simulink model "20240109_HVDCMMCInterconnection"  (R2023b)
settings: Solver=FixedStepDiscrete  StartTime=0.0  StopTime=2  FixedStep=Ts_Power  RelTol=1e-4  EnableMultiTasking=on
PreLoadFcn:
  | HVDCMMCInterconnectionParam
StartFcn:
  | tic
StopFcn:
  | toc
values from neighbouring files (symbols this model uses):
  C_PM = 1.758e-3    (= 0.001758)    [HVDCMMCInterconnectionParam.m]
  Cg = 50e-9    (= 5e-08)    [HVDCMMCInterconnectionParam.m]
  D_R = 0.001    [HVDCMMCInterconnectionParam.m]
  D_Rs = 1e8    (= 100000000)    [HVDCMMCInterconnectionParam.m]
  D_Vf = 0    [HVDCMMCInterconnectionParam.m]
  Fnom = 50    [HVDCMMCInterconnectionParam.m]
  HRM = 2    [HVDCMMCInterconnectionParam.m]
  Ki_Ireg = 6    [HVDCMMCInterconnectionParam.m]
  Ki_Preg = 1.0    (= 1)    [HVDCMMCInterconnectionParam.m]
  Ki_Qreg = 1.0    (= 1)    [HVDCMMCInterconnectionParam.m]
  Ki_VDCreg = 100    [HVDCMMCInterconnectionParam.m]
  Kp_Ireg = 0.6    [HVDCMMCInterconnectionParam.m]
  Kp_Preg = 0.5/3    (= 0.166666666667)    [HVDCMMCInterconnectionParam.m]
  Kp_Qreg = 0.5/3    (= 0.166666666667)    [HVDCMMCInterconnectionParam.m]
  Kp_VDCreg = 4    [HVDCMMCInterconnectionParam.m]
  L_cable = 15e-3    (= 0.015)    [HVDCMMCInterconnectionParam.m]
  Larm = Larm_pu*(Zb_ac/(2*pi*Fnom))    [HVDCMMCInterconnectionParam.m]
  Lff = Larm_pu/2    (= 0.075)    [HVDCMMCInterconnectionParam.m]
  Limits_Ireg = [ 2.0  -2.0]    [HVDCMMCInterconnectionParam.m]
  Limits_Preg = [ 1.2, 0.8 ]    [HVDCMMCInterconnectionParam.m]
  Limits_Qreg = [ 0.25, -0.25 ]    [HVDCMMCInterconnectionParam.m]
  Limits_VDCreg = [ 2.0  -2.0]    [HVDCMMCInterconnectionParam.m]
  Lxfo = 0.12    [HVDCMMCInterconnectionParam.m]
  Nb_PM = 36    [HVDCMMCInterconnectionParam.m]
  Pnom = 1000e6    (= 1000000000)    [HVDCMMCInterconnectionParam.m]
  R_cable = 0.5    [HVDCMMCInterconnectionParam.m]
  R_startup = 400    [HVDCMMCInterconnectionParam.m]
  Rarm = Rarm_pu*Zb_ac    [HVDCMMCInterconnectionParam.m]
  Rff = Rarm_pu/2    (= 0.00075)    [HVDCMMCInterconnectionParam.m]
  Rg = 100    [HVDCMMCInterconnectionParam.m]
  Rxfo = 0.003    [HVDCMMCInterconnectionParam.m]
  Slope_Pref = 0.5    [HVDCMMCInterconnectionParam.m]
  Slope_Qref = 0.5    [HVDCMMCInterconnectionParam.m]
  Slope_Vdc_ref = Vnom_dc/5    (= 128000)    [HVDCMMCInterconnectionParam.m]
  Tbrk1_On = 0.1    [HVDCMMCInterconnectionParam.m]
  Tbrk2_On = 1.0    (= 1)    [HVDCMMCInterconnectionParam.m]
  Tdeblock = 1.5    [HVDCMMCInterconnectionParam.m]
  Tfault = 9999    [HVDCMMCInterconnectionParam.m]
  Ton_Converter2 = 4    [HVDCMMCInterconnectionParam.m]
  Ton_PQreg = 4    [HVDCMMCInterconnectionParam.m]
  Ton_VDCreg = 1.5    [HVDCMMCInterconnectionParam.m]
  Ts = Ts_Control    (= 4e-05)    [HVDCMMCInterconnectionParam.m]
  Ts_Control = 40e-6    (= 4e-05)    [HVDCMMCInterconnectionParam.m]
  Ts_Power = 20e-6    (= 2e-05)    [HVDCMMCInterconnectionParam.m]
  Vb_ac = sqrt(2/3)*Vnom_sec    [HVDCMMCInterconnectionParam.m]
  Vb_dc = Vnom_dc    (= 640000)    [HVDCMMCInterconnectionParam.m]
  Vc0_PM = 0    [HVDCMMCInterconnectionParam.m]
  Vnom_dc = 640e3    (= 640000)    [HVDCMMCInterconnectionParam.m]
  Vnom_prim = 400e3    (= 400000)    [HVDCMMCInterconnectionParam.m]
  Vnom_sec = 333e3    (= 333000)    [HVDCMMCInterconnectionParam.m]
  w = 2*pi*Fnom    (= 314.159265359)    [HVDCMMCInterconnectionParam.m]
undefined symbols (not defined in the file or in its folder): DiscIntNeverNeededParam, gcbh, Pcc, S, sps_AC, sps_ACDC2, sps_rtmsupport
libraries: simulink x48, spsControlledVoltageSourceLib x30, spsCurrentMeasurementLib x30, MMC_Lib x30, spsDiodeLib x20, spsSeriesRLCBranchLib x14, powerlib_extras x12, spsVoltageMeasurementLib x12, spsSecondOrderFilterLib x8, spsabctodq0Lib x8, spsGroundLib x7, spsMeanLib x4
(part 5 of 9)

== system 20240109_HVDCMMCInterconnection/Model ==
  Uswitch : Inport
  status : Inport  Port=2
  0 1 : Constant  Value=0
  Gain : Gain  Gain=1./D_R  SaturateOnIntegerOverflow=on  OutDataTypeStr=Inherit: Same as input  ParamDataTypeStr=Inherit: Same as input
  Saturation : Saturate  UpperLimit=inf  LowerLimit=0
  Sum : Sum  Inputs=|++  InputSameDT=on  SaturateOnIntegerOverflow=on  OutDataTypeStr=Inherit: Same as first input
  Switch : Switch  Threshold=0.5  SaturateOnIntegerOverflow=off
  eee : Constant  Value=D_Vf
  iSwitch : Outport
  vf : Outport  Port=2
  wires:
  Uswitch/1 -> Gain/1, Sum/1
  Gain/1 -> Switch/1
  0 1/1 -> Switch/3
  Switch/1 -> Saturation/1
  eee/1 -> Sum/2, vf/1
  Saturation/1 -> iSwitch/1
  status/1 -> Switch/2

== system 20240109_HVDCMMCInterconnection/Model1 ==
  Uswitch : Inport
  status : Inport  Port=2
  0 1 : Constant  Value=0
  Gain : Gain  Gain=1./D_R  SaturateOnIntegerOverflow=on  OutDataTypeStr=Inherit: Same as input  ParamDataTypeStr=Inherit: Same as input
  Saturation : Saturate  UpperLimit=inf  LowerLimit=0
  Switch : Switch  Threshold=0.5  SaturateOnIntegerOverflow=off
  iSwitch : Outport
  wires:
  Uswitch/1 -> Gain/1
  Gain/1 -> Switch/1
  0 1/1 -> Switch/3
  Switch/1 -> Saturation/1
  Saturation/1 -> iSwitch/1
  status/1 -> Switch/2

== system 20240109_HVDCMMCInterconnection/Model2 ==
  Uswitch : Inport
  status : Inport  Port=2
  0 1 : Constant  Value=0
  Gain : Gain  Gain=1./D_R  SaturateOnIntegerOverflow=on  OutDataTypeStr=Inherit: Same as input  ParamDataTypeStr=Inherit: Same as input
  Saturation : Saturate  UpperLimit=inf  LowerLimit=0
  Switch : Switch  Threshold=0.5  SaturateOnIntegerOverflow=off
  iSwitch : Outport
  wires:
  Uswitch/1 -> Gain/1
  Gain/1 -> Switch/1
  0 1/1 -> Switch/3
  Switch/1 -> Saturation/1
  Saturation/1 -> iSwitch/1
  status/1 -> Switch/2

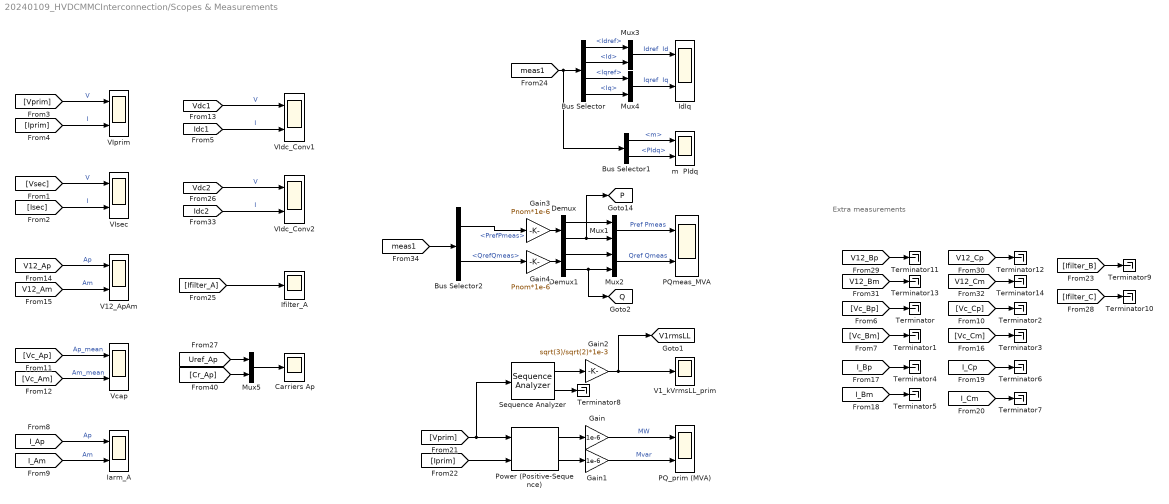
== system 20240109_HVDCMMCInterconnection/Scopes & Measurements ==
  note: Extra measurements
  Bus Selector : BusSelector  OutputSignals=Idref,Id,Iqref,Iq
  Bus Selector1 : BusSelector  OutputSignals=m,PIdq
  Bus Selector2 : BusSelector  OutputSignals=PrefPmeas,QrefQmeas
  Carriers Ap : Scope
  Demux : Demux  Outputs=2
  Demux1 : Demux  Outputs=2
  Gain : Gain  Gain=1e-6
  Gain1 : Gain  Gain=1e-6
  Gain2 : Gain  Gain=sqrt(3)/sqrt(2)*1e-3
  Gain3 : Gain  Gain=Pnom*1e-6
  Gain4 : Gain  Gain=Pnom*1e-6
  Iarm_A : Scope  NumInputPorts=2
  IdIq : Scope  NumInputPorts=2
  Ifilter_A : Scope
  Mux{1..5} (5 alike) : Mux  Inputs=2
  PQ_prim (MVA) : Scope  NumInputPorts=2
  PQmeas_MVA : Scope  NumInputPorts=2
  Power (Positive-Sequence) : spsPowerPositiveSequenceLib/Power (Positive-Sequence)  Freq=Fnom  Vinit=[0, 0]  Iinit=[0, 0]  Ts=Ts_Power
  Sequence Analyzer : spsSequenceAnalyzerLib/Sequence Analyzer  Freq=Fnom  n=1  seq=Positive  InInit=[1, 0]  Ts=Ts_Power
  Terminator{,1..14} (15 alike) : Terminator
  V12_ApAm : Scope  NumInputPorts=2
  V1_kVrmsLL_prim : Scope
  VIdc_Conv1 : Scope  NumInputPorts=2
  VIdc_Conv2 : Scope  NumInputPorts=2
  VIprim : Scope  NumInputPorts=2
  VIsec : Scope  NumInputPorts=2
  Vcap : Scope  NumInputPorts=2
  m  PIdq : Scope  NumInputPorts=2
  tag scope: P=global, Q=global, V1rmsLL=global
  wires:
  Mux5/1 -> Carriers Ap/1
  [Cr_Ap] -> Mux5/2
  [Uref_Ap] -> Mux5/1
  [Vc_Am] -> Vcap/2  "Am_mean"
  [Vc_Ap] -> Vcap/1  "Ap_mean"
  [Idc2] -> VIdc_Conv2/2  "I"
  [Vdc2] -> VIdc_Conv2/1  "V"
  Gain4/1 -> Demux1/1
  Gain3/1 -> Demux/1
  Mux2/1 -> PQmeas_MVA/2  "Qref Qmeas"
  Bus Selector2/2 -> Gain4/1  "<QrefQmeas>"
  Bus Selector2/1 -> Gain3/1  "<PrefPmeas>"
  Mux1/1 -> PQmeas_MVA/1  "Pref Pmeas"
  [meas1] -> Bus Selector2/1
  Gain2/1 -> V1_kVrmsLL_prim/1, [V1rmsLL]
  Gain1/1 -> PQ_prim (MVA)/2  "Mvar"
  Gain/1 -> PQ_prim (MVA)/1  "MW"
  [V12_Cm] -> Terminator14/1
  [V12_Bm] -> Terminator13/1
  [V12_Cp] -> Terminator12/1
  [V12_Bp] -> Terminator11/1
  [Ifilter_C] -> Terminator10/1
  [Ifilter_B] -> Terminator9/1
  Sequence Analyzer/1 -> Gain2/1
  Power (Positive-Sequence)/2 -> Gain1/1
  Power (Positive-Sequence)/1 -> Gain/1
  Sequence Analyzer/2 -> Terminator8/1
  [Iprim] -> Power (Positive-Sequence)/2
  [Vprim] -> Power (Positive-Sequence)/1, Sequence Analyzer/1
  [Idc1] -> VIdc_Conv1/2  "I"
  [Vdc1] -> VIdc_Conv1/1  "V"
  [Ifilter_A] -> Ifilter_A/1
  Bus Selector/4 -> Mux4/2  "<Iq>"
  Bus Selector/3 -> Mux4/1  "<Iqref>"
  Bus Selector/2 -> Mux3/2  "<Id>"
  Bus Selector/1 -> Mux3/1  "<Idref>"
  Mux4/1 -> IdIq/2  "Iqref  Iq"
  Mux3/1 -> IdIq/1  "Idref  Id"
  Bus Selector1/2 -> m  PIdq/2  "<PIdq>"
  Bus Selector1/1 -> m  PIdq/1  "<m>"
  [meas1] -> Bus Selector/1, Bus Selector1/1
  [I_Cm] -> Terminator7/1
  [I_Cp] -> Terminator6/1
  [I_Bm] -> Terminator5/1
  [I_Bp] -> Terminator4/1
  [I_Am] -> Iarm_A/2  "Am"
  [I_Ap] -> Iarm_A/1  "Ap"
  [Vc_Cm] -> Terminator3/1
  [Vc_Cp] -> Terminator2/1
  [Vc_Bm] -> Terminator1/1
  [Vc_Bp] -> Terminator/1
  [V12_Am] -> V12_ApAm/2  "Am"
  [V12_Ap] -> V12_ApAm/1  "Ap"
  [Vsec] -> VIsec/1  "V"
  [Isec] -> VIsec/2  "I"
  [Vprim] -> VIprim/1  "V"
  [Iprim] -> VIprim/2  "I"
  Demux/1 -> Mux1/1
  Demux/2 -> [P], Mux1/2
  Demux1/1 -> Mux2/1
  Demux1/2 -> [Q], Mux2/2

== system 20240109_HVDCMMCInterconnection/Sequencer ==
  note: Open breaker 1 when a fault occur
  note: Block the converter when a fault occur
  note: Block the converter when a fault occur
  note: STEP 6: Reactive power regulator setpoint
  note: STEP 4: Enable PQ regulators and converter 2
  note: STEP 5: Active power regulator setpoint
  note: STEP 3 : Voltage regulator setpoint
  note: STEP 2 : Deblocking converter 1
  note: STEP 1 : Energization
  note: EXTRA STEP: Program a fault
  BL1 : Step  Time=Tbrk1_On  SampleTime=Ts_Power
  BL10 : Step  Time=Tfault+Ts_Power  SampleTime=Ts_Power
  BL11 : Step  Time=Tfault  SampleTime=Ts_Power
  BL2 : Step  Time=Tbrk2_On  SampleTime=Ts_Power
  BL3 : Step  Time=Ton_Converter2  SampleTime=Ts_Power
  BL4 : Step  Time=Ton_VDCreg  SampleTime=Ts
  BL5 : Step  Time=Tdeblock  Before=1  After=0  SampleTime=Ts_Power
  BL6 : Step  Time=Ton_PQreg  SampleTime=Ts
  BL8 : Step  Time=Tfault + 1.95*(1/Fnom)  Before=1  After=0  SampleTime=Ts_Power
  BL9 : Step  Time=Tfault + 2*(1/Fnom)  Before=1  After=0  SampleTime=Ts_Power
  Logical Operator : Logic  AllPortsSameDT=off  OutDataTypeStr=boolean
  Logical Operator1 : Logic  Operator=OR  AllPortsSameDT=off  OutDataTypeStr=float('double')
  Logical Operator2 : Logic  AllPortsSameDT=off  OutDataTypeStr=boolean
  Pref : simulink/Sources/Ramp  slope=Slope_Pref  start=Tramping_Pref  InitialOutput=0
  Qref : simulink/Sources/Ramp  slope=Slope_Qref  start=Tramping_Qref  InitialOutput=0
  Rate Transition3 : RateTransition  OutPortSampleTime=Ts_Control
  Rate Transition4 : RateTransition  OutPortSampleTime=Ts_Control
  Rate Transition5 : RateTransition  OutPortSampleTime=Ts_Control
  Saturation : Saturate  UpperLimit=1  LowerLimit=-1
  Saturation1 : Saturate  UpperLimit=Limits_Qreg(1)  LowerLimit=Limits_Qreg(2)
  Saturation2 : Saturate  UpperLimit=Vnom_dc  LowerLimit=eps
  "Vdc_ref " : simulink/Sources/Ramp  slope=Slope_Vdc_ref  start=Tramping_Vdc_ref  InitialOutput=Vnom_sec*1.37
  tag scope: Blk=global, Brk1_On=global, Brk2_On=global, Converter2_On=global, Fault_On=global, PQreg_On=global, Pref=global, Qref=global, VDCreg_On=global, Vdc_ref=global
  wires:
  Saturation2/1 -> Rate Transition5/1
  Saturation1/1 -> Rate Transition4/1
  Pref/1 -> Saturation/1
  Qref/1 -> Saturation1/1
  Saturation/1 -> Rate Transition3/1
  Rate Transition3/1 -> [Pref]
  Rate Transition4/1 -> [Qref]
  Rate Transition5/1 -> [Vdc_ref]
  BL4/1 -> [VDCreg_On]
  BL6/1 -> [PQreg_On]
  "Vdc_ref "/1 -> Saturation2/1
  BL2/1 -> [Brk2_On]
  BL8/1 -> Logical Operator/2
  Logical Operator/1 -> [Brk1_On]
  BL1/1 -> Logical Operator/1
  BL9/1 -> Logical Operator2/2
  BL3/1 -> Logical Operator2/1
  Logical Operator2/1 -> [Converter2_On]
  Logical Operator1/1 -> [Blk]
  BL5/1 -> Logical Operator1/1
  BL10/1 -> Logical Operator1/2
  BL11/1 -> [Fault_On]

== system 20240109_HVDCMMCInterconnection/Sources ==
  3ph SM1 : Subsystem
  3ph SM2 : Subsystem
  3ph SM3 : Subsystem
  3ph SM4 : Subsystem
  3ph SM5 : Subsystem
  3ph SM6 : Subsystem
  Demux : Demux  Outputs=3
  From1 : From  Commented=on  GotoTag=T60_5595_6094221501797  TagVisibility=global
  From10 : From  Commented=on  GotoTag=Bp_Vbl_EMT  TagVisibility=global
  From11 : From  Commented=on  GotoTag=Bp_Vin_EMT  TagVisibility=global
  From12 : From  Commented=on  GotoTag=Cn_Vbl_EMT  TagVisibility=global
  From13 : From  Commented=on  GotoTag=Cn_Vin_EMT  TagVisibility=global
  From14 : From  Commented=on  GotoTag=Cp_Vbl_EMT  TagVisibility=global
  From15 : From  Commented=on  GotoTag=Cp_Vin_EMT  TagVisibility=global
  From16 : From  Commented=on  GotoTag=An_Vbl_EMT  TagVisibility=global
  From17 : From  Commented=on  GotoTag=An_Vin_EMT  TagVisibility=global
  From2 : From  Commented=on  GotoTag=T61_5644_6069908417486  TagVisibility=global
  From4 : From  Commented=on  GotoTag=An_Vbl_EMT  TagVisibility=global
  From5 : From  Commented=on  GotoTag=An_Vin_EMT  TagVisibility=global
  From6 : From  Commented=on  GotoTag=Ap_Vbl_EMT  TagVisibility=global
  From7 : From  Commented=on  GotoTag=Ap_Vin_EMT  TagVisibility=global
  From8 : From  Commented=on  GotoTag=Bn_Vbl_EMT  TagVisibility=global
  From9 : From  Commented=on  GotoTag=Bn_Vin_EMT  TagVisibility=global
  Mux : Mux  Inputs=[1 1 1 1 1 1 1 1 1 1 1 1 1 1 1 1 1]
  Mux1 : Mux  Commented=on  Inputs=2
  Mux2 : Mux  Commented=on  Inputs=2
  Mux_u : Mux  Inputs=[14 17]
  Scope : Scope  Commented=on  NumInputPorts=2
  Scope1 : Scope  NumInputPorts=2
  SwitchCurrents : Constant  Value=zeros(14,1)
  u : Outport  VectorParamsAs1DForOutWhenUnconnected=off
  wires:
  Mux_u/1 -> u/1
  SwitchCurrents/1 -> Mux_u/1
  Mux/1 -> Mux_u/2
  From1/1 -> Scope1/1, Mux/1
  From2/1 -> Scope1/2, Mux/2
  3ph SM1/1(An_Vbl) -> Mux/3
  3ph SM1/2(An_Vin) -> Mux/4
  3ph SM2/1(An_Vbl) -> Mux/5
  3ph SM2/2(An_Vin) -> Mux/6
  3ph SM3/1(An_Vbl) -> Mux/7
  3ph SM3/2(An_Vin) -> Mux/8
  3ph SM4/1(An_Vbl) -> Mux/9
  3ph SM4/2(An_Vin) -> Mux/10
  3ph SM5/1(An_Vbl) -> Mux/11
  3ph SM5/2(An_Vin) -> Mux/12
  3ph SM6/1(An_Vbl) -> Mux/13
  Demux/1 -> Mux/15
  Demux/2 -> Mux/16
  Demux/3 -> Mux/17
  [Vsrc_ABC] -> Demux/1
  3ph SM6/2(An_Vin) -> Mux/14
  [SF_An_Icap] -> 3ph SM1/3(An_Icap)
  [SF_An_Ipos] -> 3ph SM1/2(An_Ipos)
  [Uref_An_sf] -> 3ph SM1/1(Uref_An)
  From16/1 -> Mux1/1
  Mux2/1 -> Scope/2
  ? -> Mux1/2
  Mux1/1 -> Scope/1
  ? -> Mux2/2
  From17/1 -> Mux2/1
  [Uref_Ap_sf] -> 3ph SM2/1(Uref_An)
  [SF_Ap_Ipos] -> 3ph SM2/2(An_Ipos)
  [SF_Ap_Icap] -> 3ph SM2/3(An_Icap)
  [SF_Bp_Icap] -> 3ph SM4/3(An_Icap)
  [SF_Bp_Ipos] -> 3ph SM4/2(An_Ipos)
  [Uref_Bn_sf] -> 3ph SM3/1(Uref_An)
  [Uref_Bp_sf] -> 3ph SM4/1(Uref_An)
  [SF_Bn_Ipos] -> 3ph SM3/2(An_Ipos)
  [SF_Bn_Icap] -> 3ph SM3/3(An_Icap)
  [SF_Cp_Icap] -> 3ph SM6/3(An_Icap)
  [SF_Cp_Ipos] -> 3ph SM6/2(An_Ipos)
  [Uref_Cn_sf] -> 3ph SM5/1(Uref_An)
  [Uref_Cp_sf] -> 3ph SM6/1(Uref_An)
  [SF_Cn_Ipos] -> 3ph SM5/2(An_Ipos)
  [SF_Cn_Icap] -> 3ph SM5/3(An_Icap)

== system 20240109_HVDCMMCInterconnection/Sources1 ==
  3ph SM1 : Subsystem
  3ph SM2 : Subsystem
  3ph SM3 : Subsystem
  3ph SM4 : Subsystem
  3ph SM5 : Subsystem
  3ph SM6 : Subsystem
  Demux : Demux  Outputs=3
  From2 : From  Commented=on  GotoTag=T61_5644_6069908417486  TagVisibility=global
  Mux : Mux  Inputs=[1 1 1 1 1 1 1 1 1 1 1 1 1 1 1 1 1]
  Mux_u : Mux  Inputs=[14 17]
  Scope1 : Scope  NumInputPorts=2
  SwitchCurrents : Constant  Value=zeros(14,1)
  u : Outport  VectorParamsAs1DForOutWhenUnconnected=off
  wires:
  Mux_u/1 -> u/1
  SwitchCurrents/1 -> Mux_u/1
  Mux/1 -> Mux_u/2
  [Vdc2t] -> Mux/1
  [Vdc2b] -> Mux/2
  3ph SM1/1(An_Vbl) -> Scope1/2, Mux/3, Scope1/1
  3ph SM1/2(An_Vin) -> Mux/4
  3ph SM2/1(An_Vbl) -> Mux/5
  3ph SM2/2(An_Vin) -> Mux/6
  3ph SM3/1(An_Vbl) -> Mux/7
  3ph SM3/2(An_Vin) -> Mux/8
  3ph SM4/1(An_Vbl) -> Mux/9
  3ph SM4/2(An_Vin) -> Mux/10
  3ph SM5/1(An_Vbl) -> Mux/11
  3ph SM5/2(An_Vin) -> Mux/12
  3ph SM6/1(An_Vbl) -> Mux/13
  Demux/1 -> Mux/15
  Demux/2 -> Mux/16
  Demux/3 -> Mux/17
  [Vsrc_ABC] -> Demux/1
  3ph SM6/2(An_Vin) -> Mux/14
  [SF_An_Icap1] -> 3ph SM1/3(An_Icap)
  [SF_An_Ipos1] -> 3ph SM1/2(An_Ipos)
  [Uref_An_sf1] -> 3ph SM1/1(Uref_An)
  [Uref_Ap_sf1] -> 3ph SM2/1(Uref_An)
  [SF_Ap_Ipos1] -> 3ph SM2/2(An_Ipos)
  [SF_Ap_Icap1] -> 3ph SM2/3(An_Icap)
  [SF_Bp_Icap1] -> 3ph SM4/3(An_Icap)
  [SF_Bp_Ipos1] -> 3ph SM4/2(An_Ipos)
  [Uref_Bn_sf1] -> 3ph SM3/1(Uref_An)
  [Uref_Bp_sf1] -> 3ph SM4/1(Uref_An)
  [SF_Bn_Ipos1] -> 3ph SM3/2(An_Ipos)
  [SF_Bn_Icap1] -> 3ph SM3/3(An_Icap)
  [SF_Cp_Icap1] -> 3ph SM6/3(An_Icap)
  [SF_Cp_Ipos1] -> 3ph SM6/2(An_Ipos)
  [Uref_Cn_sf1] -> 3ph SM5/1(Uref_An)
  [Uref_Cp_sf1] -> 3ph SM6/1(Uref_An)
  [SF_Cn_Ipos1] -> 3ph SM5/2(An_Ipos)
  [SF_Cn_Icap1] -> 3ph SM5/3(An_Icap)

== system 20240109_HVDCMMCInterconnection/Status1 ==
  status : Inport
  Demux : Demux  Outputs=[1 1 1 1 1 1 1 1 1 1 1 1 1 1]
  Gain : Gain  Gain=0
  Goto1 : Goto  Commented=on  GotoTag=T49_4510_4258244859575
  Goto10 : Goto  Commented=on  GotoTag=T42_3788_2930675327927  TagVisibility=global
  Goto11 : Goto  Commented=on  GotoTag=T42_3768_2824731541533  TagVisibility=global
  Goto12 : Goto  Commented=on  GotoTag=T42_3786_2916524331498  TagVisibility=global
  Goto13 : Goto  Commented=on  GotoTag=T42_3772_2839034668200  TagVisibility=global
  Goto14 : Goto  Commented=on  GotoTag=T42_3790_2930678723391  TagVisibility=global
  Goto2 : Goto  Commented=on  GotoTag=T50_4559_4296145620637
  Goto3 : Goto  Commented=on  GotoTag=T42_3764_2824687999628
  Goto4 : Goto  Commented=on  GotoTag=T42_3782_2916624610639  TagVisibility=global
  Goto5 : Goto  Commented=on  GotoTag=T42_3768_2839018950081  TagVisibility=global
  Goto6 : Goto  Commented=on  GotoTag=T43_3835_2986319703090  TagVisibility=global
  Goto7 : Goto  Commented=on  GotoTag=T42_3766_2824642323653  TagVisibility=global
  Goto8 : Goto  Commented=on  GotoTag=T42_3784_2916507024141  TagVisibility=global
  Goto9 : Goto  Commented=on  GotoTag=T42_3770_2838959362213  TagVisibility=global
  Scope : Scope
  wires:
  status/1 -> Scope/1, Gain/1
  Demux/1 -> Goto1/1
  Demux/2 -> Goto2/1
  Demux/3 -> Goto3/1
  Demux/4 -> Goto4/1
  Demux/5 -> Goto5/1
  Demux/6 -> Goto6/1
  Demux/7 -> Goto7/1
  Demux/8 -> Goto8/1
  Demux/9 -> Goto9/1
  Demux/10 -> Goto10/1
  Demux/11 -> Goto11/1
  Demux/12 -> Goto12/1
  Demux/13 -> Goto13/1
  Demux/14 -> Goto14/1
  Gain/1 -> Demux/1

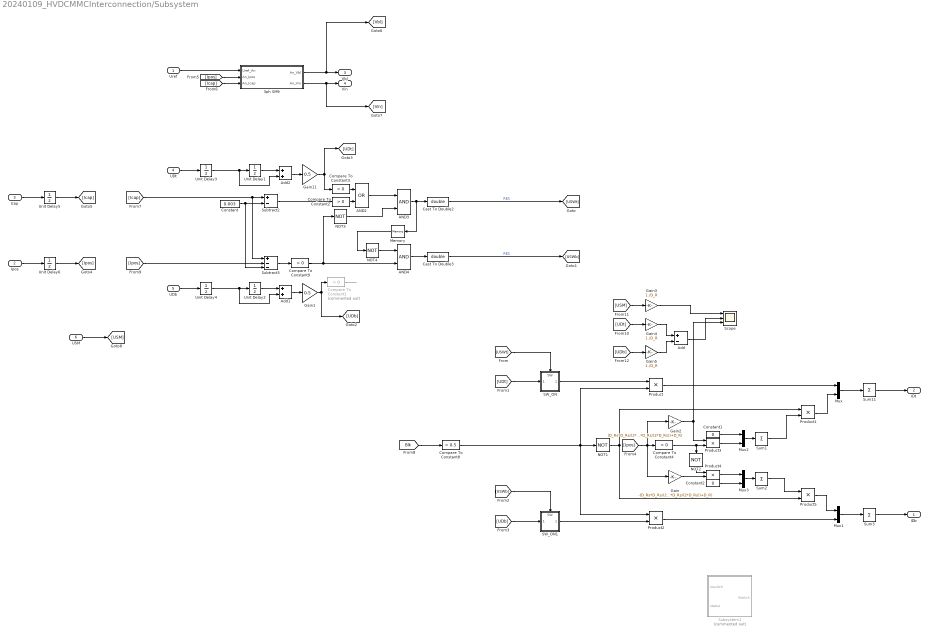
== system 20240109_HVDCMMCInterconnection/Subsystem ==
  Uref : Inport
  Ipos : Inport  Port=2
  Icap : Inport  Port=3
  UDt : Inport  Port=4
  UDb : Inport  Port=5
  USM : Inport  Port=6
  3ph SM9 : Subsystem
  AND2 : Logic  Operator=OR  IconShape=distinctive  AllPortsSameDT=off  OutDataTypeStr=boolean
  AND3 : Logic  IconShape=distinctive  AllPortsSameDT=off  OutDataTypeStr=boolean
  AND4 : Logic  IconShape=distinctive  AllPortsSameDT=off  OutDataTypeStr=boolean
  Add : Sum  Inputs=+-
  Add1 : Sum
  Add2 : Sum
  Cast To Double2 : DataTypeConversion  OutDataTypeStr=double  SaturateOnIntegerOverflow=off  RndMeth=Floor
  Cast To Double3 : DataTypeConversion  OutDataTypeStr=double  SaturateOnIntegerOverflow=off  RndMeth=Floor
  Compare To Constant1 : simulink/Logic and Bit Operations/Compare To Constant  Commented=on  relop=>  const=0  OutDataTypeStr=boolean
  Compare To Constant{2..4,9} (4 alike) : simulink/Logic and Bit Operations/Compare To Constant  relop=>  const=0  OutDataTypeStr=boolean
  Compare To Constant8 : simulink/Logic and Bit Operations/Compare To Constant  relop=>  const=0.5  OutDataTypeStr=boolean
  Constant : Constant  Value=0.003
  Constant1 : Constant  Value=0
  Constant2 : Constant  Value=0
  Gain : Gain  Gain=-(D_Rs*D_Rs/(2*D_Rs))/((D_Rs*D_Rs/(2*D_Rs))+D_R)
  Gain1 : Gain  Gain=0.5
  Gain11 : Gain  Gain=0.5
  Gain2 : Gain  Gain=(D_Rs*D_Rs/(2*D_Rs))/((D_Rs*D_Rs/(2*D_Rs))+D_R)
  Gain3 : Gain  Gain=1./D_R
  Gain4 : Gain  Gain=1./D_R
  Gain5 : Gain  Gain=1./D_R
  Memory : Memory
  Mux{,1..3} (4 alike) : Mux  Inputs=2
  NOT{1..4} (4 alike) : Logic  Operator=NOT  IconShape=distinctive  AllPortsSameDT=off  OutDataTypeStr=boolean
  Product{,1..5} (6 alike) : Product
  SW_ON : Subsystem
      settings: PortSchema="{\"entries\":[{\"content\":{\"sides\":[{\"content\":{\"connectorIds\":[\"In1\"]},\"type\":\"ConnectorPlacement.EquallySpacedRectSide\",\"uuid\":\"61570b56-e5d0-4812-b143-8fea08408b82\"},{\"content\":{\"connectorIds\":[\"Out1\"],\"side\":\"RIGHT\"},\"type\":\"ConnectorPlacement.EquallySpacedRectSide\",\"uuid\":\"fb1b449d-dcf0-4498-bfcd-c35d1b8d3af1\"},{\"content\":{\"connectorIds\":[\"In2\"],\"side\":\"TOP\"},\"type\":\"ConnectorPlacement.EquallySpacedRectSide\",\"uuid\":\"2091de1c-d6a0-4f6b-9728-c6eb9657220b\"}]},\"type\":\"ConnectorPlacement.EquallySpacedConnector\",\"uuid\":\"fce121a6-5cfd-4a9e-88a9-d62df4eca96b\"}],\"packageUris\":[\"http://schema.mathworks.com/mf0/Connector/R2020b\"],\"version\":\"1.0\"}"
  SW_ON1 : Subsystem
      settings: PortSchema="{\"entries\":[{\"content\":{\"sides\":[{\"content\":{\"connectorIds\":[\"In1\"]},\"type\":\"ConnectorPlacement.EquallySpacedRectSide\",\"uuid\":\"61570b56-e5d0-4812-b143-8fea08408b82\"},{\"content\":{\"connectorIds\":[\"Out1\"],\"side\":\"RIGHT\"},\"type\":\"ConnectorPlacement.EquallySpacedRectSide\",\"uuid\":\"fb1b449d-dcf0-4498-bfcd-c35d1b8d3af1\"},{\"content\":{\"connectorIds\":[\"In2\"],\"side\":\"TOP\"},\"type\":\"ConnectorPlacement.EquallySpacedRectSide\",\"uuid\":\"2091de1c-d6a0-4f6b-9728-c6eb9657220b\"}]},\"type\":\"ConnectorPlacement.EquallySpacedConnector\",\"uuid\":\"fce121a6-5cfd-4a9e-88a9-d62df4eca96b\"}],\"packageUris\":[\"http://schema.mathworks.com/mf0/Connector/R2020b\"],\"version\":\"1.0\"}"
  Scope : Scope  NumInputPorts=3
  Subsystem1 : Subsystem  Commented=on
  Subtract2 : Sum  Inputs=+-
  Subtract3 : Sum  Inputs=+--
  Sum{1..3,11} (4 alike) : Sum  Inputs=1  InputSameDT=on  SaturateOnIntegerOverflow=on  OutDataTypeStr=Inherit: Same as first input
  Unit Delay{1..6} (6 alike) : UnitDelay  SampleTime=Ts_Power  HasFrameUpgradeWarning=on
  IDb : Outport
  IDt : Outport  Port=2
  Vbl : Outport  Port=3
  Vin : Outport  Port=4
  wires:
  Unit Delay4/1 -> Unit Delay2/1, Add1/2
  Unit Delay3/1 -> Unit Delay1/1, Add2/2
  Unit Delay6/1 -> [Ipos]
  [Ipos] -> Subtract3/2
  Unit Delay5/1 -> [Icap]
  [Icap] -> Subtract2/1, Subtract3/1
  3ph SM9/2(An_Vin) -> Vin/1, [Vin]
  3ph SM9/1(An_Vbl) -> Vbl/1, [Vbl]
  Uref/1 -> 3ph SM9/1(Uref_An)
  [Icap] -> 3ph SM9/3(An_Icap)
  [Ipos] -> 3ph SM9/2(An_Ipos)
  Constant1/1 -> Mux2/1
  Gain2/1 -> Scope/3, Product3/1
  Sum3/1 -> IDb/1
  Gain/1 -> Product4/2
  NOT2/1 -> Product4/1
  Product5/1 -> Mux1/1
  Constant2/1 -> Mux3/2
  Sum2/1 -> Product5/1
  Mux3/1 -> Sum2/1
  Product4/1 -> Mux3/1
  Compare To Constant4/1 -> Product3/2, NOT2/1
  [Ipos] -> Gain/1, Compare To Constant4/1, Gain2/1
  Sum1/1 -> Product1/2
  Product3/1 -> Mux2/2
  Mux2/1 -> Sum1/1
  Mux/1 -> Sum11/1
  Sum11/1 -> IDt/1
  Mux1/1 -> Sum3/1
  Product2/1 -> Mux1/2
  SW_ON1/1(Out1) -> Product2/2
  Product1/1 -> Mux/2
  NOT1/1 -> Product5/2, Product1/1
  Product/1 -> Mux/1
  SW_ON/1(Out1) -> Product/1
  Compare To Constant8/1 -> Product2/1, NOT1/1, Product/2
  [Blk] -> Compare To Constant8/1
  [USWb] -> SW_ON1/2(SW)
  [UDb] -> SW_ON1/1(In1)
  [UDt] -> SW_ON/1(In1)
  [USWt] -> SW_ON/2(SW)
  Compare To Constant1/1 -> ?
  Gain1/1 -> Compare To Constant1/1, [UDb]
  Add1/1 -> Gain1/1
  Unit Delay2/1 -> Add1/1
  UDb/1 -> Unit Delay4/1
  Compare To Constant9/1 -> NOT3/1, AND4/2
  Memory/1 -> NOT4/1
  Icap/1 -> Unit Delay5/1
  AND4/1 -> Cast To Double3/1
  Cast To Double3/1 -> [USWb]  "RES"
  Compare To Constant2/1 -> AND2/2
  AND3/1 -> Memory/1, Cast To Double2/1
  Subtract2/1 -> Compare To Constant2/1
  Subtract3/1 -> Compare To Constant9/1
  Cast To Double2/1 -> [USWt]  "RES"
  Add2/1 -> Gain11/1
  Unit Delay1/1 -> Add2/1
  Compare To Constant3/1 -> AND2/1
  Gain11/1 -> Compare To Constant3/1, [UDt]
  NOT3/1 -> AND3/2
  AND2/1 -> AND3/1
  NOT4/1 -> AND4/1
  Ipos/1 -> Unit Delay6/1
  Constant/1 -> Subtract2/2, Subtract3/3
  UDt/1 -> Unit Delay3/1
  [USM] -> Gain3/1
  USM/1 -> [USM]
  [UDt] -> Gain4/1
  [UDb] -> Gain5/1
  Gain4/1 -> Add/1
  Gain5/1 -> Add/2
  Add/1 -> Scope/2
  Gain3/1 -> Scope/1

== system 20240109_HVDCMMCInterconnection/Uref2m1 ==
  In1 : Inport
  Add1 : Sum
  Compare To Constant1 : simulink/Logic and Bit Operations/Compare To Constant  relop=<=  const=0.5  OutDataTypeStr=boolean
  Compare To Constant2 : simulink/Logic and Bit Operations/Compare To Constant  relop=<=  const=0.5  OutDataTypeStr=boolean
  Constant6 : Constant
  Constant7 : Constant  Value=0
  Constant9 : Constant
  Gain3 : Gain  Gain=0.5
  Mux : Mux  Inputs=2
  Saturation1 : Saturate  UpperLimit=1  LowerLimit=0
  Switch1 : Switch  Criteria=u2 ~= 0  SaturateOnIntegerOverflow=off  InputSameDT=off
  Switch2 : Switch  Criteria=u2 ~= 0  SaturateOnIntegerOverflow=off  InputSameDT=off
  Uref : Outport
  wires:
  Switch1/1 -> Mux/1
  [Blk] -> Compare To Constant1/1, Compare To Constant2/1
  Add1/1 -> Gain3/1
  Gain3/1 -> Switch1/1
  Constant7/1 -> Switch1/3, Switch2/1
  Compare To Constant1/1 -> Switch2/2
  Constant6/1 -> Add1/2
  Mux/1 -> Saturation1/1
  Constant9/1 -> Switch2/3
  Compare To Constant2/1 -> Switch1/2
  Switch2/1 -> Mux/2
  In1/1 -> Add1/1
  Saturation1/1 -> Uref/1

== system 20240109_HVDCMMCInterconnection/Uref2m2 ==
  Uref_ABC : Inport  PortDimensions=3
  Block : Inport  Port=2
  Add1 : Sum
  Add2 : Sum
  Compare To Constant{1..4} (4 alike) : simulink/Logic and Bit Operations/Compare To Constant  relop=<=  const=0.5  OutDataTypeStr=boolean
  Constant1 : Constant
  Constant2 : Constant  Value=[0 0 0]
  Constant3 : Constant  Value=[1 1 1]
  Constant6 : Constant
  Constant7 : Constant  Value=[0 0 0]
  Constant9 : Constant  Value=[1 1 1]
  Demux{,2..4} (4 alike) : Demux  Outputs=3
  Gain1 : Gain  Gain=-1
  Gain2 : Gain  Gain=0.5
  Gain3 : Gain  Gain=0.5
  Mux{,1..2,4..6} (6 alike) : Mux  Inputs=2
  Saturation{1,3..5} (4 alike) : Saturate  UpperLimit=1  LowerLimit=0
  Switch{1..4} (4 alike) : Switch  Criteria=u2 ~= 0  SaturateOnIntegerOverflow=off  InputSameDT=off
  Uref_Ap : Outport
  Uref_Bp : Outport  Port=2
  Uref_Cp : Outport  Port=3
  Uref_An : Outport  Port=4
  Uref_Bn : Outport  Port=5
  Uref_Cn : Outport  Port=6
  wires:
  Add1/1 -> Gain3/1
  Gain3/1 -> Switch1/1
  Constant7/1 -> Switch1/3, Switch2/1
  Compare To Constant1/1 -> Switch2/2
  Constant6/1 -> Add1/2
  Constant9/1 -> Switch2/3
  Compare To Constant2/1 -> Switch1/2
  Gain1/1 -> Add1/1
  Mux/1 -> Uref_Ap/1
  Switch1/1 -> Saturation1/1
  Switch2/1 -> Saturation3/1
  Demux/1 -> Mux/1
  Demux2/1 -> Mux/2
  Demux/2 -> Mux1/1
  Demux2/2 -> Mux1/2
  Demux2/3 -> Mux2/2
  Demux/3 -> Mux2/1
  Demux4/1 -> Mux4/2
  Demux4/2 -> Mux5/2
  Constant1/1 -> Add2/2
  Compare To Constant4/1 -> Switch3/2
  Compare To Constant3/1 -> Switch4/2
  Add2/1 -> Gain2/1
  Constant2/1 -> Switch3/3, Switch4/1
  Block/1 -> Compare To Constant1/1, Compare To Constant4/1, Compare To Constant3/1, Compare To Constant2/1
  Uref_ABC/1 -> Add2/1, Gain1/1
  Switch3/1 -> Saturation4/1
  Demux3/2 -> Mux5/1
  Demux3/3 -> Mux6/1
  Constant3/1 -> Switch4/3
  Demux3/1 -> Mux4/1
  Switch4/1 -> Saturation5/1
  Gain2/1 -> Switch3/1
  Demux4/3 -> Mux6/2
  Saturation1/1 -> Demux/1
  Saturation3/1 -> Demux2/1
  Saturation4/1 -> Demux3/1
  Saturation5/1 -> Demux4/1
  Mux1/1 -> Uref_Bp/1
  Mux2/1 -> Uref_Cp/1
  Mux4/1 -> Uref_An/1
  Mux5/1 -> Uref_Bn/1
  Mux6/1 -> Uref_Cn/1

== system 20240109_HVDCMMCInterconnection/Uref2m3 ==
  Uref_ABC : Inport  PortDimensions=3
  Block : Inport  Port=2
  Add1 : Sum
  Add2 : Sum
  Compare To Constant{1..4} (4 alike) : simulink/Logic and Bit Operations/Compare To Constant  relop=<=  const=0.5  OutDataTypeStr=boolean
  Constant1 : Constant
  Constant2 : Constant  Value=[0 0 0]
  Constant3 : Constant  Value=[1 1 1]
  Constant6 : Constant
  Constant7 : Constant  Value=[0 0 0]
  Constant9 : Constant  Value=[1 1 1]
  Demux{,2..4} (4 alike) : Demux  Outputs=3
  Gain1 : Gain  Gain=-1
  Gain2 : Gain  Gain=0.5
  Gain3 : Gain  Gain=0.5
  Mux{,1..2,4..6} (6 alike) : Mux  Inputs=2
  Saturation{1,3..5} (4 alike) : Saturate  UpperLimit=1  LowerLimit=0
  Switch{1..4} (4 alike) : Switch  Criteria=u2 ~= 0  SaturateOnIntegerOverflow=off  InputSameDT=off
  Uref_Ap : Outport
  Uref_Bp : Outport  Port=2
  Uref_Cp : Outport  Port=3
  Uref_An : Outport  Port=4
  Uref_Bn : Outport  Port=5
  Uref_Cn : Outport  Port=6
  wires:
  Add1/1 -> Gain3/1
  Gain3/1 -> Switch1/1
  Constant7/1 -> Switch1/3, Switch2/1
  Compare To Constant1/1 -> Switch2/2
  Constant6/1 -> Add1/2
  Constant9/1 -> Switch2/3
  Compare To Constant2/1 -> Switch1/2
  Gain1/1 -> Add1/1
  Mux/1 -> Uref_Ap/1
  Switch1/1 -> Saturation1/1
  Switch2/1 -> Saturation3/1
  Demux/1 -> Mux/1
  Demux2/1 -> Mux/2
  Demux/2 -> Mux1/1
  Demux2/2 -> Mux1/2
  Demux2/3 -> Mux2/2
  Demux/3 -> Mux2/1
  Demux4/1 -> Mux4/2
  Demux4/2 -> Mux5/2
  Constant1/1 -> Add2/2
  Compare To Constant4/1 -> Switch3/2
  Compare To Constant3/1 -> Switch4/2
  Add2/1 -> Gain2/1
  Constant2/1 -> Switch3/3, Switch4/1
  Block/1 -> Compare To Constant1/1, Compare To Constant4/1, Compare To Constant3/1, Compare To Constant2/1
  Uref_ABC/1 -> Add2/1, Gain1/1
  Switch3/1 -> Saturation4/1
  Demux3/2 -> Mux5/1
  Demux3/3 -> Mux6/1
  Constant3/1 -> Switch4/3
  Demux3/1 -> Mux4/1
  Switch4/1 -> Saturation5/1
  Gain2/1 -> Switch3/1
  Demux4/3 -> Mux6/2
  Saturation1/1 -> Demux/1
  Saturation3/1 -> Demux2/1
  Saturation4/1 -> Demux3/1
  Saturation5/1 -> Demux4/1
  Mux1/1 -> Uref_Bp/1
  Mux2/1 -> Uref_Cp/1
  Mux4/1 -> Uref_An/1
  Mux5/1 -> Uref_Bn/1
  Mux6/1 -> Uref_Cn/1

== system 20240109_HVDCMMCInterconnection/Uref2m4 ==
  Uref_ABC : Inport  PortDimensions=3
  Block : Inport  Port=2
  Add1 : Sum
  Add2 : Sum
  Compare To Constant{1..4} (4 alike) : simulink/Logic and Bit Operations/Compare To Constant  relop=<=  const=0.5  OutDataTypeStr=boolean
  Constant1 : Constant
  Constant2 : Constant  Value=[0 0 0]
  Constant3 : Constant  Value=[1 1 1]
  Constant6 : Constant
  Constant7 : Constant  Value=[0 0 0]
  Constant9 : Constant  Value=[1 1 1]
  Demux{,2..4} (4 alike) : Demux  Outputs=3
  Gain1 : Gain  Gain=-1
  Gain2 : Gain  Gain=0.5
  Gain3 : Gain  Gain=0.5
  Mux{,1..2,4..6} (6 alike) : Mux  Inputs=2
  Saturation{1,3..5} (4 alike) : Saturate  UpperLimit=1  LowerLimit=0
  Switch{1..4} (4 alike) : Switch  Criteria=u2 ~= 0  SaturateOnIntegerOverflow=off  InputSameDT=off
  Uref_Ap : Outport
  Uref_Bp : Outport  Port=2
  Uref_Cp : Outport  Port=3
  Uref_An : Outport  Port=4
  Uref_Bn : Outport  Port=5
  Uref_Cn : Outport  Port=6
  wires:
  Add1/1 -> Gain3/1
  Gain3/1 -> Switch1/1
  Constant7/1 -> Switch1/3, Switch2/1
  Compare To Constant1/1 -> Switch2/2
  Constant6/1 -> Add1/2
  Constant9/1 -> Switch2/3
  Compare To Constant2/1 -> Switch1/2
  Gain1/1 -> Add1/1
  Mux/1 -> Uref_Ap/1
  Switch1/1 -> Saturation1/1
  Switch2/1 -> Saturation3/1
  Demux/1 -> Mux/1
  Demux2/1 -> Mux/2
  Demux/2 -> Mux1/1
  Demux2/2 -> Mux1/2
  Demux2/3 -> Mux2/2
  Demux/3 -> Mux2/1
  Demux4/1 -> Mux4/2
  Demux4/2 -> Mux5/2
  Constant1/1 -> Add2/2
  Compare To Constant4/1 -> Switch3/2
  Compare To Constant3/1 -> Switch4/2
  Add2/1 -> Gain2/1
  Constant2/1 -> Switch3/3, Switch4/1
  Block/1 -> Compare To Constant1/1, Compare To Constant4/1, Compare To Constant3/1, Compare To Constant2/1
  Uref_ABC/1 -> Add2/1, Gain1/1
  Switch3/1 -> Saturation4/1
  Demux3/2 -> Mux5/1
  Demux3/3 -> Mux6/1
  Constant3/1 -> Switch4/3
  Demux3/1 -> Mux4/1
  Switch4/1 -> Saturation5/1
  Gain2/1 -> Switch3/1
  Demux4/3 -> Mux6/2
  Saturation1/1 -> Demux/1
  Saturation3/1 -> Demux2/1
  Saturation4/1 -> Demux3/1
  Saturation5/1 -> Demux4/1
  Mux1/1 -> Uref_Bp/1
  Mux2/1 -> Uref_Cp/1
  Mux4/1 -> Uref_An/1
  Mux5/1 -> Uref_Bn/1
  Mux6/1 -> Uref_Cn/1

== system 20240109_HVDCMMCInterconnection/Voltage source ==
  In1 : Inport
  Demux9 : Demux  Outputs=3
  Ground : spsGroundLib/Ground  LConnTagsString=a
  VSRC_a : spsControlledVoltageSourceLib/Controlled Voltage Source  Initialize=on  Source_Type=AC  Amplitude=0  Phase=0  Frequency=0  Measurements=None
  VSRC_b : spsControlledVoltageSourceLib/Controlled Voltage Source  Initialize=on  Source_Type=AC  Amplitude=0  Phase=0  Frequency=0  Measurements=None
  VSRC_c : spsControlledVoltageSourceLib/Controlled Voltage Source  Initialize=on  Source_Type=AC  Amplitude=0  Phase=0  Frequency=0  Measurements=None
  a : PMIOPort  Side=Right
  b : PMIOPort  Port=2  Side=Right
  c : PMIOPort  Port=3  Side=Right
  wires:
  In1/1 -> Demux9/1
  Demux9/1 -> VSRC_a/1
  Demux9/2 -> VSRC_b/1
  Demux9/3 -> VSRC_c/1
  connections:
  Ground/LConn1 -- VSRC_b/LConn1 -- VSRC_a/LConn1 -- VSRC_c/LConn1
  VSRC_c/RConn1 -- c/RConn1
  VSRC_b/RConn1 -- b/RConn1
  VSRC_a/RConn1 -- a/RConn1

== system 20240109_HVDCMMCInterconnection/Voltage source1 ==
  In1 : Inport
  Controlled Voltage Source : spsControlledVoltageSourceLib/Controlled Voltage Source  Initialize=on  Source_Type=AC  Amplitude=0  Phase=0  Frequency=0  Measurements=None
  Controlled Voltage Source6 : spsControlledVoltageSourceLib/Controlled Voltage Source  Initialize=on  Source_Type=AC  Amplitude=0  Phase=0  Frequency=0  Measurements=None
  Controlled Voltage Source7 : spsControlledVoltageSourceLib/Controlled Voltage Source  Initialize=on  Source_Type=AC  Amplitude=0  Phase=0  Frequency=0  Measurements=None
  Demux9 : Demux  Outputs=3
  Ground : spsGroundLib/Ground  LConnTagsString=a
  a : PMIOPort  Side=Right
  b : PMIOPort  Port=2  Side=Right
  c : PMIOPort  Port=3  Side=Right
  wires:
  In1/1 -> Demux9/1
  Demux9/1 -> Controlled Voltage Source/1
  Demux9/2 -> Controlled Voltage Source6/1
  Demux9/3 -> Controlled Voltage Source7/1
  connections:
  Ground/LConn1 -- Controlled Voltage Source6/LConn1 -- Controlled Voltage Source/LConn1 -- Controlled Voltage Source7/LConn1
  Controlled Voltage Source7/RConn1 -- c/RConn1
  Controlled Voltage Source6/RConn1 -- b/RConn1
  Controlled Voltage Source/RConn1 -- a/RConn1

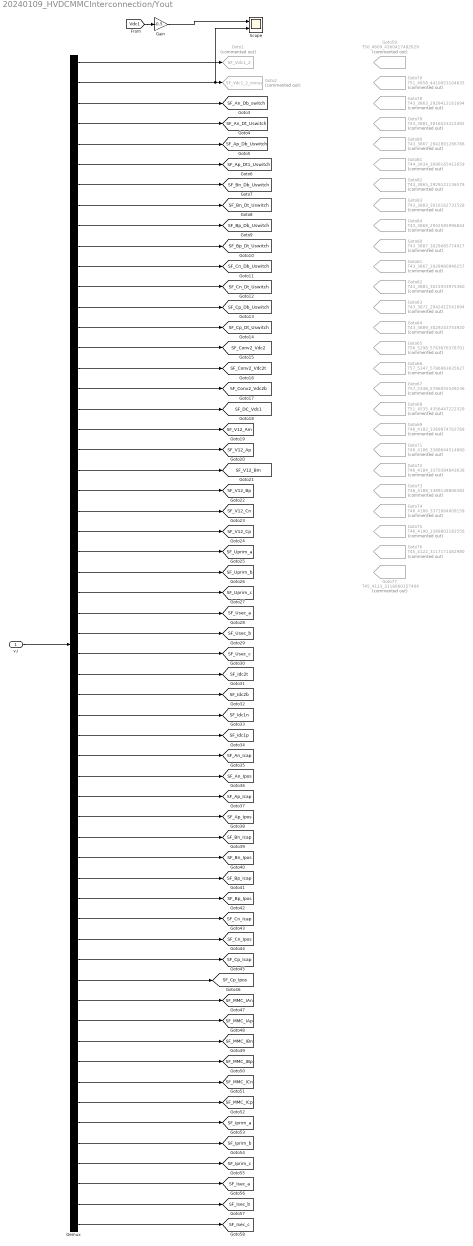
== system 20240109_HVDCMMCInterconnection/Yout ==
  v,i : Inport
  Demux : Demux  Outputs=[1 1 1 1 1 1 1 1 1 1 1 1 1 1 1 1 1 1 1 1 1 1 1 1 1 1 1 1 1 1 1 1 1 1 1 1 1 1 1 1 1 1 1 1 1 1 1 1 1 1 1 1 1 1 1 1 1 1]
  Gain : Gain  Gain=-0.5
  Goto1 : Goto  Commented=on  GotoTag=SF_Vdc1_2  TagVisibility=global
  Goto2 : Goto  Commented=on  GotoTag=SF_Vdc1_2_minus  TagVisibility=global
  Goto59 : Goto  Commented=on  GotoTag=T50_4609_4360417482629  TagVisibility=global
  Goto60 : Goto  Commented=on  GotoTag=T43_3887_3029485774917  TagVisibility=global
  Goto61 : Goto  Commented=on  GotoTag=T43_3867_2928960946257  TagVisibility=global
  Goto62 : Goto  Commented=on  GotoTag=T43_3885_3015933975360  TagVisibility=global
  Goto63 : Goto  Commented=on  GotoTag=T43_3871_2942412541694  TagVisibility=global
  Goto64 : Goto  Commented=on  GotoTag=T43_3889_3029243753920  TagVisibility=global
  Goto65 : Goto  Commented=on  GotoTag=T56_5298_5763676378701  TagVisibility=global
  Goto66 : Goto  Commented=on  GotoTag=T57_5347_5786963635627  TagVisibility=global
  Goto67 : Goto  Commented=on  GotoTag=T57_5348_5786055549236  TagVisibility=global
  Goto68 : Goto  Commented=on  GotoTag=T51_4535_4356447222329  TagVisibility=global
  Goto69 : Goto  Commented=on  GotoTag=T46_4182_3369874763768  TagVisibility=global
  Goto70 : Goto  Commented=on  GotoTag=T51_4658_4410053104635  TagVisibility=global
  Goto71 : Goto  Commented=on  GotoTag=T46_4186_3388644514860  TagVisibility=global
  Goto72 : Goto  Commented=on  GotoTag=T46_4184_3370384843638  TagVisibility=global
  Goto73 : Goto  Commented=on  GotoTag=T46_4188_3389138806382  TagVisibility=global
  Goto74 : Goto  Commented=on  GotoTag=T46_4186_3371064009159  TagVisibility=global
  Goto75 : Goto  Commented=on  GotoTag=T46_4190_3389802183556  TagVisibility=global
  Goto76 : Goto  Commented=on  GotoTag=T45_4122_3117171482980  TagVisibility=global
  Goto77 : Goto  Commented=on  GotoTag=T45_4123_3118060157404  TagVisibility=global
  Goto78 : Goto  Commented=on  GotoTag=T43_3863_2929413161694  TagVisibility=global
  Goto79 : Goto  Commented=on  GotoTag=T43_3881_3016523322492  TagVisibility=global
  Goto80 : Goto  Commented=on  GotoTag=T43_3867_2942891286788  TagVisibility=global
  Goto81 : Goto  Commented=on  GotoTag=T44_3934_3096165412659  TagVisibility=global
  Goto82 : Goto  Commented=on  GotoTag=T43_3865_2929121136578  TagVisibility=global
  Goto83 : Goto  Commented=on  GotoTag=T43_3883_3016162731528  TagVisibility=global
  Goto84 : Goto  Commented=on  GotoTag=T43_3869_2942585996844  TagVisibility=global
  Scope : Scope  NumInputPorts=2
  tag scope: SF_An_Db_switch=global, SF_An_Dt_Uswitch=global, SF_An_Icap=global, SF_An_Ipos=global, SF_Ap_Db_Uswitch=global, SF_Ap_Dt1_Uswitch=global, SF_Ap_Icap=global, SF_Ap_Ipos=global, SF_Bn_Db_Uswitch=global, SF_Bn_Dt_Uswitch=global, SF_Bn_Icap=global, SF_Bn_Ipos=global, SF_Bp_Db_Uswitch=global, SF_Bp_Dt_Uswitch=global, SF_Bp_Icap=global, SF_Bp_Ipos=global, SF_Cn_Db_Uswitch=global, SF_Cn_Dt_Uswitch=global, SF_Cn_Icap=global, SF_Cn_Ipos=global, SF_Conv2_Vdc2=global, SF_Conv2_Vdc2b=global, SF_Conv2_Vdc2t=global, SF_Cp_Db_Uswitch=global, SF_Cp_Dt_Uswitch=global, SF_Cp_Icap=global, SF_Cp_Ipos=global, SF_DC_Vdc1=global, SF_Idc1n=global, SF_Idc1p=global, SF_Idc2b=global, SF_Idc2t=global, SF_Iprim_a=global, SF_Iprim_b=global, SF_Iprim_c=global, SF_Isec_a=global, SF_Isec_b=global, SF_Isec_c=global, SF_MMC_IAn=global, SF_MMC_IAp=global, SF_MMC_IBn=global, SF_MMC_IBp=global, SF_MMC_ICn=global, SF_MMC_ICp=global, SF_Uprim_a=global, SF_Uprim_b=global, SF_Uprim_c=global, SF_Usec_a=global, SF_Usec_b=global, SF_Usec_c=global, SF_V12_Am=global, SF_V12_Ap=global, SF_V12_Bm=global, SF_V12_Bp=global, SF_V12_Cn=global, SF_V12_Cp=global
  wires:
  v,i/1 -> Demux/1
  Demux/1 -> Goto1/1
  Demux/2 -> Scope/2, Goto2/1
  Demux/3 -> [SF_An_Db_switch]
  Demux/4 -> [SF_An_Dt_Uswitch]
  Demux/5 -> [SF_Ap_Db_Uswitch]
  Demux/6 -> [SF_Ap_Dt1_Uswitch]
  Demux/7 -> [SF_Bn_Db_Uswitch]
  Demux/8 -> [SF_Bn_Dt_Uswitch]
  Demux/9 -> [SF_Bp_Db_Uswitch]
  Demux/10 -> [SF_Bp_Dt_Uswitch]
  Demux/11 -> [SF_Cn_Db_Uswitch]
  Demux/12 -> [SF_Cn_Dt_Uswitch]
  Demux/13 -> [SF_Cp_Db_Uswitch]
  Demux/14 -> [SF_Cp_Dt_Uswitch]
  Demux/15 -> [SF_Conv2_Vdc2]
  Demux/16 -> [SF_Conv2_Vdc2t]
  Demux/17 -> [SF_Conv2_Vdc2b]
  Demux/18 -> [SF_DC_Vdc1]
  Demux/19 -> [SF_V12_Am]
  Demux/20 -> [SF_V12_Ap]
  Demux/21 -> [SF_V12_Bm]
  Demux/22 -> [SF_V12_Bp]
  Demux/23 -> [SF_V12_Cn]
  Demux/24 -> [SF_V12_Cp]
  Demux/25 -> [SF_Uprim_a]
  Demux/26 -> [SF_Uprim_b]
  Demux/27 -> [SF_Uprim_c]
  Demux/28 -> [SF_Usec_a]
  Demux/29 -> [SF_Usec_b]
  Demux/30 -> [SF_Usec_c]
  Demux/31 -> [SF_Idc2t]
  Demux/32 -> [SF_Idc2b]
  Demux/33 -> [SF_Idc1n]
  Demux/34 -> [SF_Idc1p]
  Demux/35 -> [SF_An_Icap]
  Demux/36 -> [SF_An_Ipos]
  Demux/37 -> [SF_Ap_Icap]
  Demux/38 -> [SF_Ap_Ipos]
  Demux/39 -> [SF_Bn_Icap]
  Demux/40 -> [SF_Bn_Ipos]
  Demux/41 -> [SF_Bp_Icap]
  Demux/42 -> [SF_Bp_Ipos]
  Demux/43 -> [SF_Cn_Icap]
  Demux/44 -> [SF_Cn_Ipos]
  Demux/45 -> [SF_Cp_Icap]
  Demux/46 -> [SF_Cp_Ipos]
  Demux/47 -> [SF_MMC_IAn]
  Demux/48 -> [SF_MMC_IAp]
  Demux/49 -> [SF_MMC_IBn]
  Demux/50 -> [SF_MMC_IBp]
  Demux/51 -> [SF_MMC_ICn]
  Demux/52 -> [SF_MMC_ICp]
  Demux/53 -> [SF_Iprim_a]
  Demux/54 -> [SF_Iprim_b]
  Demux/55 -> [SF_Iprim_c]
  Demux/56 -> [SF_Isec_a]
  Demux/57 -> [SF_Isec_b]
  Demux/58 -> [SF_Isec_c]
  [Vdc1] -> Gain/1
  Gain/1 -> Scope/1

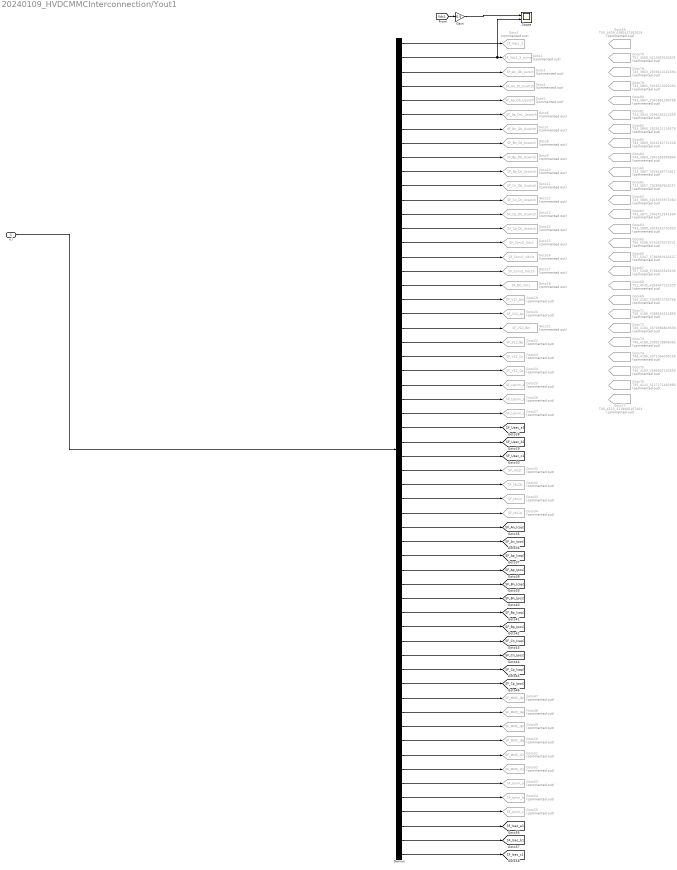
== system 20240109_HVDCMMCInterconnection/Yout1 ==
  v,i : Inport
  Demux : Demux  Outputs=[1 1 1 1 1 1 1 1 1 1 1 1 1 1 1 1 1 1 1 1 1 1 1 1 1 1 1 1 1 1 1 1 1 1 1 1 1 1 1 1 1 1 1 1 1 1 1 1 1 1 1 1 1 1 1 1 1 1]
  Gain : Gain  Gain=-0.5
  Goto1 : Goto  Commented=on  GotoTag=SF_Vdc1_2  TagVisibility=global
  Goto10 : Goto  Commented=on  GotoTag=SF_Bp_Dt_Uswitch  TagVisibility=global
  Goto11 : Goto  Commented=on  GotoTag=SF_Cn_Db_Uswitch  TagVisibility=global
  Goto12 : Goto  Commented=on  GotoTag=SF_Cn_Dt_Uswitch  TagVisibility=global
  Goto13 : Goto  Commented=on  GotoTag=SF_Cp_Db_Uswitch  TagVisibility=global
  Goto14 : Goto  Commented=on  GotoTag=SF_Cp_Dt_Uswitch  TagVisibility=global
  Goto15 : Goto  Commented=on  GotoTag=SF_Conv2_Vdc2  TagVisibility=global
  Goto16 : Goto  Commented=on  GotoTag=SF_Conv2_Vdc2t  TagVisibility=global
  Goto17 : Goto  Commented=on  GotoTag=SF_Conv2_Vdc2b  TagVisibility=global
  Goto18 : Goto  Commented=on  GotoTag=SF_DC_Vdc1  TagVisibility=global
  Goto19 : Goto  Commented=on  GotoTag=SF_V12_Am  TagVisibility=global
  Goto2 : Goto  Commented=on  GotoTag=SF_Vdc1_2_minus  TagVisibility=global
  Goto20 : Goto  Commented=on  GotoTag=SF_V12_Ap  TagVisibility=global
  Goto21 : Goto  Commented=on  GotoTag=SF_V12_Bm  TagVisibility=global
  Goto22 : Goto  Commented=on  GotoTag=SF_V12_Bp  TagVisibility=global
  Goto23 : Goto  Commented=on  GotoTag=SF_V12_Cn  TagVisibility=global
  Goto24 : Goto  Commented=on  GotoTag=SF_V12_Cp  TagVisibility=global
  Goto25 : Goto  Commented=on  GotoTag=SF_Uprim_a  TagVisibility=global
  Goto26 : Goto  Commented=on  GotoTag=SF_Uprim_b  TagVisibility=global
  Goto27 : Goto  Commented=on  GotoTag=SF_Uprim_c  TagVisibility=global
  Goto3 : Goto  Commented=on  GotoTag=SF_An_Db_switch  TagVisibility=global
  Goto31 : Goto  Commented=on  GotoTag=SF_Idc2t  TagVisibility=global
  Goto32 : Goto  Commented=on  GotoTag=SF_Idc2b  TagVisibility=global
  Goto33 : Goto  Commented=on  GotoTag=SF_Idc1n  TagVisibility=global
  Goto34 : Goto  Commented=on  GotoTag=SF_Idc1p  TagVisibility=global
  Goto4 : Goto  Commented=on  GotoTag=SF_An_Dt_Uswitch  TagVisibility=global
  Goto47 : Goto  Commented=on  GotoTag=SF_MMC_IAn  TagVisibility=global
  Goto48 : Goto  Commented=on  GotoTag=SF_MMC_IAp  TagVisibility=global
  Goto49 : Goto  Commented=on  GotoTag=SF_MMC_IBn  TagVisibility=global
  Goto5 : Goto  Commented=on  GotoTag=SF_Ap_Db_Uswitch  TagVisibility=global
  Goto50 : Goto  Commented=on  GotoTag=SF_MMC_IBp  TagVisibility=global
  Goto51 : Goto  Commented=on  GotoTag=SF_MMC_ICn  TagVisibility=global
  Goto52 : Goto  Commented=on  GotoTag=SF_MMC_ICp  TagVisibility=global
  Goto53 : Goto  Commented=on  GotoTag=SF_Iprim_a  TagVisibility=global
  Goto54 : Goto  Commented=on  GotoTag=SF_Iprim_b  TagVisibility=global
  Goto55 : Goto  Commented=on  GotoTag=SF_Iprim_c  TagVisibility=global
  Goto59 : Goto  Commented=on  GotoTag=T50_4609_4360417482629  TagVisibility=global
  Goto6 : Goto  Commented=on  GotoTag=SF_Ap_Dt1_Uswitch  TagVisibility=global
  Goto60 : Goto  Commented=on  GotoTag=T43_3887_3029485774917  TagVisibility=global
  Goto61 : Goto  Commented=on  GotoTag=T43_3867_2928960946257  TagVisibility=global
  Goto62 : Goto  Commented=on  GotoTag=T43_3885_3015933975360  TagVisibility=global
  Goto63 : Goto  Commented=on  GotoTag=T43_3871_2942412541694  TagVisibility=global
  Goto64 : Goto  Commented=on  GotoTag=T43_3889_3029243753920  TagVisibility=global
  Goto65 : Goto  Commented=on  GotoTag=T56_5298_5763676378701  TagVisibility=global
  Goto66 : Goto  Commented=on  GotoTag=T57_5347_5786963635627  TagVisibility=global
  Goto67 : Goto  Commented=on  GotoTag=T57_5348_5786055549236  TagVisibility=global
  Goto68 : Goto  Commented=on  GotoTag=T51_4535_4356447222329  TagVisibility=global
  Goto69 : Goto  Commented=on  GotoTag=T46_4182_3369874763768  TagVisibility=global
  Goto7 : Goto  Commented=on  GotoTag=SF_Bn_Db_Uswitch  TagVisibility=global
  Goto70 : Goto  Commented=on  GotoTag=T51_4658_4410053104635  TagVisibility=global
  Goto71 : Goto  Commented=on  GotoTag=T46_4186_3388644514860  TagVisibility=global
  Goto72 : Goto  Commented=on  GotoTag=T46_4184_3370384843638  TagVisibility=global
  Goto73 : Goto  Commented=on  GotoTag=T46_4188_3389138806382  TagVisibility=global
  Goto74 : Goto  Commented=on  GotoTag=T46_4186_3371064009159  TagVisibility=global
  Goto75 : Goto  Commented=on  GotoTag=T46_4190_3389802183556  TagVisibility=global
  Goto76 : Goto  Commented=on  GotoTag=T45_4122_3117171482980  TagVisibility=global
  Goto77 : Goto  Commented=on  GotoTag=T45_4123_3118060157404  TagVisibility=global
  Goto78 : Goto  Commented=on  GotoTag=T43_3863_2929413161694  TagVisibility=global
  Goto79 : Goto  Commented=on  GotoTag=T43_3881_3016523322492  TagVisibility=global
  Goto8 : Goto  Commented=on  GotoTag=SF_Bn_Dt_Uswitch  TagVisibility=global
  Goto80 : Goto  Commented=on  GotoTag=T43_3867_2942891286788  TagVisibility=global
  Goto81 : Goto  Commented=on  GotoTag=T44_3934_3096165412659  TagVisibility=global
  Goto82 : Goto  Commented=on  GotoTag=T43_3865_2929121136578  TagVisibility=global
  Goto83 : Goto  Commented=on  GotoTag=T43_3883_3016162731528  TagVisibility=global
  Goto84 : Goto  Commented=on  GotoTag=T43_3869_2942585996844  TagVisibility=global
  Goto9 : Goto  Commented=on  GotoTag=SF_Bp_Db_Uswitch  TagVisibility=global
  Scope : Scope  NumInputPorts=2
  tag scope: SF_An_Icap1=global, SF_An_Ipos1=global, SF_Ap_Icap1=global, SF_Ap_Ipos1=global, SF_Bn_Icap1=global, SF_Bn_Ipos1=global, SF_Bp_Icap1=global, SF_Bp_Ipos1=global, SF_Cn_Icap1=global, SF_Cn_Ipos1=global, SF_Cp_Icap1=global, SF_Cp_Ipos1=global, SF_Isec_a1=global, SF_Isec_b1=global, SF_Isec_c1=global, SF_Usec_a1=global, SF_Usec_b1=global, SF_Usec_c1=global
  wires:
  v,i/1 -> Demux/1
  Demux/1 -> Goto1/1
  Demux/2 -> Scope/2, Goto2/1
  Demux/3 -> Goto3/1
  Demux/4 -> Goto4/1
  Demux/5 -> Goto5/1
  Demux/6 -> Goto6/1
  Demux/7 -> Goto7/1
  Demux/8 -> Goto8/1
  Demux/9 -> Goto9/1
  Demux/10 -> Goto10/1
  Demux/11 -> Goto11/1
  Demux/12 -> Goto12/1
  Demux/13 -> Goto13/1
  Demux/14 -> Goto14/1
  Demux/15 -> Goto15/1
  Demux/16 -> Goto16/1
  Demux/17 -> Goto17/1
  Demux/18 -> Goto18/1
  Demux/19 -> Goto19/1
  Demux/20 -> Goto20/1
  Demux/21 -> Goto21/1
  Demux/22 -> Goto22/1
  Demux/23 -> Goto23/1
  Demux/24 -> Goto24/1
  Demux/25 -> Goto25/1
  Demux/26 -> Goto26/1
  Demux/27 -> Goto27/1
  Demux/28 -> [SF_Usec_a1]
  Demux/29 -> [SF_Usec_b1]
  Demux/30 -> [SF_Usec_c1]
  Demux/31 -> Goto31/1
  Demux/32 -> Goto32/1
  Demux/33 -> Goto33/1
  Demux/34 -> Goto34/1
  Demux/35 -> [SF_An_Icap1]
  Demux/36 -> [SF_An_Ipos1]
  Demux/37 -> [SF_Ap_Icap1]
  Demux/38 -> [SF_Ap_Ipos1]
  Demux/39 -> [SF_Bn_Icap1]
  Demux/40 -> [SF_Bn_Ipos1]
  Demux/41 -> [SF_Bp_Icap1]
  Demux/42 -> [SF_Bp_Ipos1]
  Demux/43 -> [SF_Cn_Icap1]
  Demux/44 -> [SF_Cn_Ipos1]
  Demux/45 -> [SF_Cp_Icap1]
  Demux/46 -> [SF_Cp_Ipos1]
  Demux/47 -> Goto47/1
  Demux/48 -> Goto48/1
  Demux/49 -> Goto49/1
  Demux/50 -> Goto50/1
  Demux/51 -> Goto51/1
  Demux/52 -> Goto52/1
  Demux/53 -> Goto53/1
  Demux/54 -> Goto54/1
  Demux/55 -> Goto55/1
  Demux/56 -> [SF_Isec_a1]
  Demux/57 -> [SF_Isec_b1]
  Demux/58 -> [SF_Isec_c1]
  [Vdc1] -> Gain/1
  Gain/1 -> Scope/1

== system 20240109_HVDCMMCInterconnection/param ==

== system 20240109_HVDCMMCInterconnection/Control/Active Power Regulator (Preg) ==
  note: Active Power Regulator
  Pmeas : Inport  PortDimensions=1
  Pref : Inport  Port=2  PortDimensions=1  SampleTime=Ts
  On : Inport  Port=3  PortDimensions=1  SampleTime=Ts
  Discrete-Time Integrator : DiscreteIntegrator  InitialCondition=1  SampleTime=Ts  LimitOutput=on  UpperSaturationLimit=Limits_Preg(1)  LowerSaturationLimit=Limits_Preg(2)  ICPrevOutput=DiscIntNeverNeededParam  ICPrevScaledInput=DiscIntNeverNeededParam
  Product : Product  RndMeth=Zero
  Product1 : Product  RndMeth=Zero
  Product2 : Product
  Saturation2 : Saturate  UpperLimit=Limits_Preg(1)  LowerLimit=Limits_Preg(2)  SampleTime=Ts
  Sum : Sum  Inputs=|+-
  Sum6 : Sum  InputSameDT=on  SaturateOnIntegerOverflow=on  SampleTime=Ts  OutDataTypeStr=Inherit: Same as first input
  Switch1 : Switch  Criteria=u2 ~= 0  Threshold=0.5  OutDataTypeStr=double  SaturateOnIntegerOverflow=off  InputSameDT=off
  VdcNom_SM : Constant  Value=Kp_Preg  SampleTime=Ts
  VdcNom_SM1 : Constant  Value=Ki_Preg  SampleTime=Ts
  VdcNom_SM2 : Constant  Value=Vnom_dc  SampleTime=Ts
  Zero-Order Hold : ZeroOrderHold  SampleTime=Ts
  Vdc_ref : Outport  SampleTime=Ts
  wires:
  Product2/1 -> Vdc_ref/1
  VdcNom_SM2/1 -> Product2/2
  Pmeas/1 -> Switch1/1
  On/1 -> Switch1/2
  Switch1/1 -> Sum/1
  Pref/1 -> Switch1/3, Sum/2
  Zero-Order Hold/1 -> Sum6/1
  Discrete-Time Integrator/1 -> Sum6/2
  Sum6/1 -> Saturation2/1
  VdcNom_SM1/1 -> Product/1
  Product1/1 -> Zero-Order Hold/1
  Product/1 -> Discrete-Time Integrator/1
  VdcNom_SM/1 -> Product1/1
  Saturation2/1 -> Product2/1
  Sum/1 -> Product1/2, Product/2
